simulink model "inner_axe"  (R2021a)
settings: Solver=VariableStepAuto  StartTime=0.0  StopTime=100.0  RelTol=1e-3
settings Model: Creator=user  LastModifiedBy=user

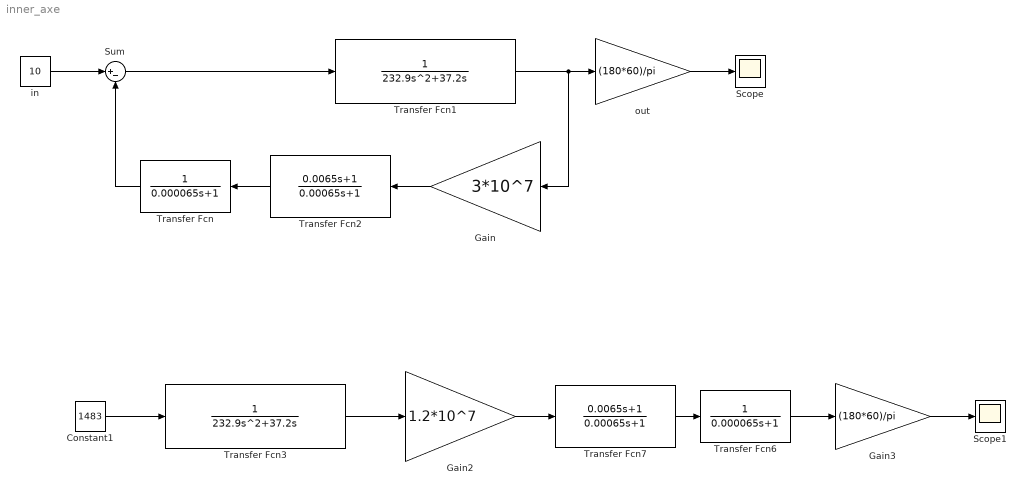
== system inner_axe ==
  Constant1 : Constant  Value=1483  SampleTime=1
  Gain : Gain  Gain=3*10^7
  Gain2 : Gain  Gain=1.2*10^7
  Gain3 : Gain  Gain=(180*60)/pi
  Scope : Scope
  Scope1 : Scope
  Sum : Sum  Inputs=|+-
  Transfer Fcn : TransferFcn  Denominator=[0.000065 1]
  Transfer Fcn1 : TransferFcn  Denominator=[232.9 37.2 0]
  Transfer Fcn2 : TransferFcn  Numerator=[0.0065 1]  Denominator=[0.00065 1]
  Transfer Fcn3 : TransferFcn  Denominator=[232.9 37.2 0]
  Transfer Fcn6 : TransferFcn  Denominator=[0.000065 1]
  Transfer Fcn7 : TransferFcn  Numerator=[0.0065 1]  Denominator=[0.00065 1]
  in : Constant  Value=10  SampleTime=1
  out : Gain  Gain=(180*60)/pi
  wires:
  Transfer Fcn1/1 -> Gain/1, out/1
  Sum/1 -> Transfer Fcn1/1
  out/1 -> Scope/1
  in/1 -> Sum/1
  Gain/1 -> Transfer Fcn2/1
  Gain3/1 -> Scope1/1
  Constant1/1 -> Transfer Fcn3/1
  Transfer Fcn3/1 -> Gain2/1
  Gain2/1 -> Transfer Fcn7/1
  Transfer Fcn/1 -> Sum/2
  Transfer Fcn2/1 -> Transfer Fcn/1
  Transfer Fcn7/1 -> Transfer Fcn6/1
  Transfer Fcn6/1 -> Gain3/1
